simulink model "ADRC_14a"  (R2014a)
settings: Solver=ode45  SolverMode=SingleTasking  StartTime=0.0  StopTime=10.0  RelTol=1e-3
model workspace (MAT data in the model file):
  b = Simulink.Parameter
  b.DataType = 'auto'
  b.Dimensions = [0 0]
  kp = Simulink.Parameter
  kp.DataType = 'auto'
  kp.Dimensions = [0 0]
settings Model: CovMetricSettings=dwe  CovHtmlReporting=off  covSaveCumulativeToWorkspaceVar=off  CovSaveSingleToWorkspaceVar=off  CovExternalEMLEnable=on  CovSFcnEnable=on  Creator=leony  LastModifiedBy=root
settings DataIOCC: LimitDataPoints=off  SaveFormat=StructureWithTime  ReturnWorkspaceOutputs=on
settings DebuggingCC: MergeDetectMultiDrivingBlocksExec=error  SolverPrmCheckMsg=none  FrameProcessingCompatibilityMsg=error  SFUnexpectedBacktrackingDiag=error  SFNoUnconditionalDefaultTransitionDiag=error
settings HardwareCC: ProdBitPerPointer=64  ProdLargestAtomicFloat=Float  ProdIntDivRoundTo=Zero  ProdEndianess=LittleEndian  ProdHWDeviceType=Specified
settings ModelReferenceCC: PropagateSignalLabelsOutOfModel=on
settings SFSimCC: SimUseLocalCustomCode=on
settings RTWCC: RTWUseLocalCustomCode=on
settings GRTTargetCC: TargetLangStandard=C99 (ISO)  GeneratePreprocessorConditionals=Use local settings

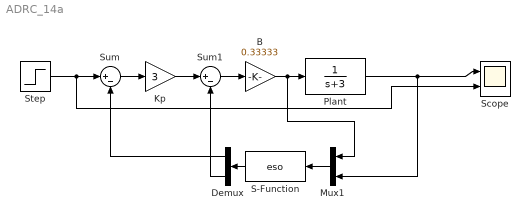
== system ADRC_14a ==
  B : Gain  Gain=0.33333  ParamDataTypeStr=double
  Demux : Demux  Outputs=2
  Kp : Gain  Gain=3
  Mux1 : Mux  Inputs=2
  Plant : TransferFcn  Numerator=1  Denominator="[1  3]"
  S-Function : S-Function  FunctionName=eso  Parameters=b, kp  SFunctionDeploymentMode=off  EnableBusSupport=off
  Scope : Scope  NumInputPorts=2
      settings: TimeRange=auto  MaxDataPoints=5000  SaveToWorkspace=off  SaveName=ScopeData  YMin=-0.125~-5  YMax=1.125~5  SampleTime=-1
  Step : Step  SampleTime=0
  Sum : Sum  Inputs=|+-
  Sum1 : Sum  Inputs=|+-
  wires:
  Plant/1 -> Mux1/2, Scope/1
  Mux1/1 -> S-Function/1
  S-Function/1 -> Demux/1
  Step/1 -> Scope/2, Sum/1
  Demux/1 -> Sum/2
  Sum/1 -> Kp/1
  Kp/1 -> Sum1/1
  Demux/2 -> Sum1/2
  Sum1/1 -> B/1
  B/1 -> Mux1/1, Plant/1
